simulink model "ex_longlat_kinematic"  (R2026a)
settings: Solver=VariableStepAuto
libraries: aerolibconvert2 x3
settings Model: Creator=doyeop  LastModifiedBy=doyeop

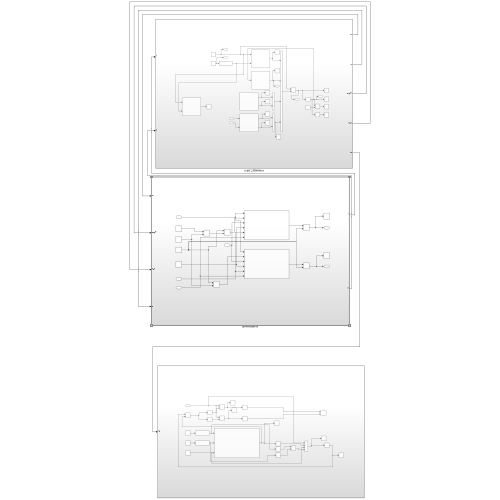
[thumbnail: Simulink's stored preview of the top-level diagram]
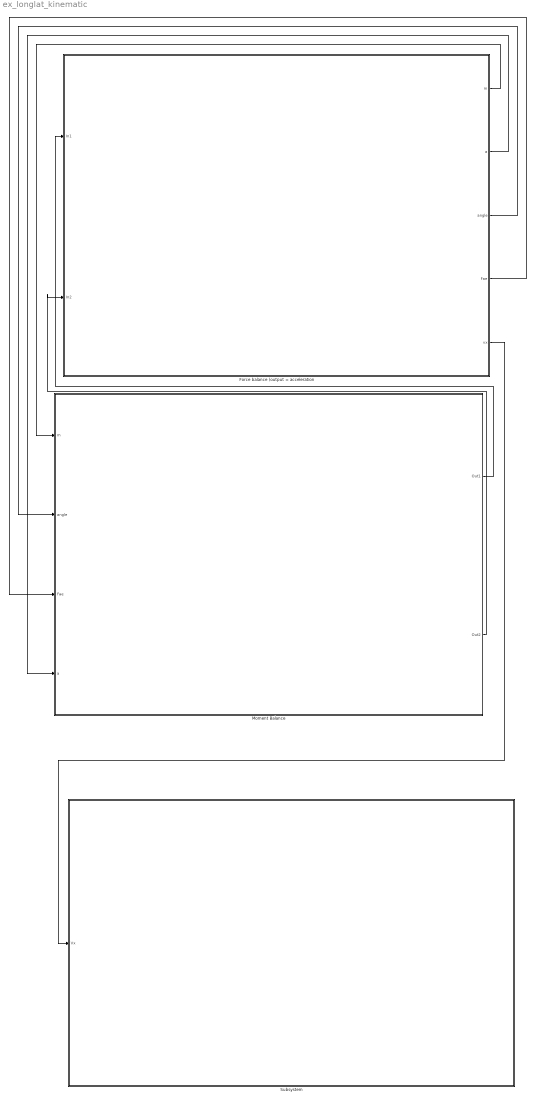
== system ex_longlat_kinematic ==
  Force balance (output = acceleration : Subsystem
  Moment Balance : Subsystem
  Subsystem : Subsystem
  wires:
  Force balance (output = acceleration/1(m) -> Moment Balance/1(m)
  Force balance (output = acceleration/2(a) -> Moment Balance/4(a)
  Force balance (output = acceleration/3(angle) -> Moment Balance/2(angle)
  Force balance (output = acceleration/4(Fae) -> Moment Balance/3(Fae)
  Moment Balance/1(Out1) -> Force balance (output = acceleration/1(In1)
  Moment Balance/2(Out2) -> Force balance (output = acceleration/2(In2)
  Force balance (output = acceleration/5(vx) -> Subsystem/1(Vx)

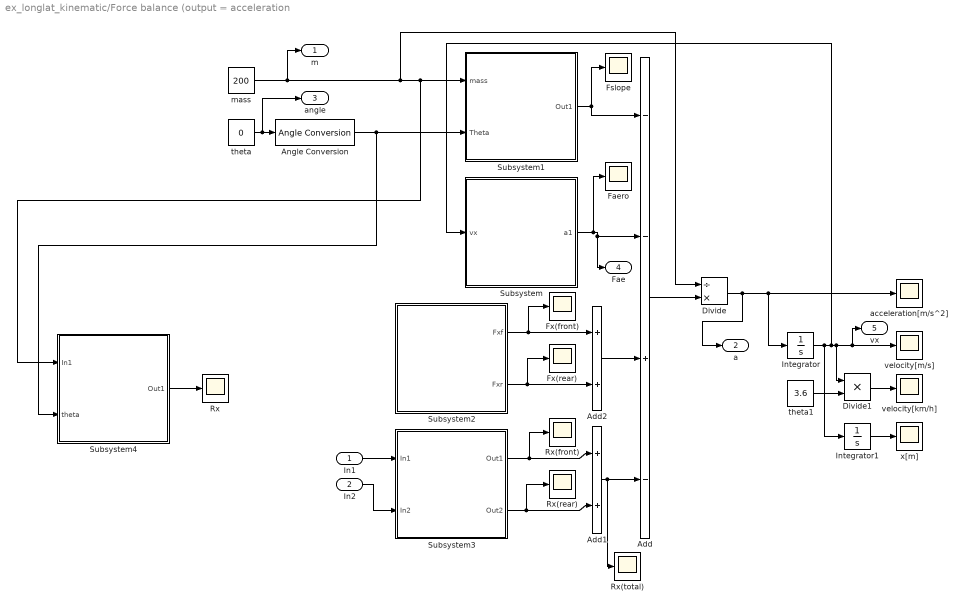
== system ex_longlat_kinematic/Force balance (output = acceleration ==
  In1 : Inport
  In2 : Inport  Port=2
  Add : Sum  Inputs=--+-
  Add1 : Sum
  Add2 : Sum
  Angle Conversion : aerolibconvert2/Angle Conversion  IU=deg  OU=rad
  Divide : Product  Inputs=/*
  Divide1 : Product  Inputs=**
  Faero : Scope
      settings: ActiveDisplayYMinimum=-21.806973838724872  ActiveDisplayYMaximum=245.93181269445461  DataLoggingVariableName=ScopeData4
  Fslope : Scope
      settings: ActiveDisplayYMinimum=467.68768501992645  ActiveDisplayYMaximum=4126.826484026702  DataLoggingVariableName=ScopeData3
  Fx(front) : Scope
      settings: ActiveDisplayYMinimum=-0.77322383064043154  ActiveDisplayYMaximum=0.91988628090500946  DataLoggingVariableName=ScopeData5
  Fx(rear) : Scope
      settings: ActiveDisplayYMinimum=-0.77322383064043154  ActiveDisplayYMaximum=0.91988628090500946  DataLoggingVariableName=ScopeData10
  Integrator : Integrator
  Integrator1 : Integrator
  Rx : Scope
      settings: ActiveDisplayYMinimum=21.392000000000003  ActiveDisplayYMaximum=41.392  DataLoggingVariableName=ScopeData6
  Rx(front) : Scope
      settings: ActiveDisplayYMinimum=-1  ActiveDisplayYMaximum=1  DataLoggingVariableName=ScopeData11
  Rx(rear) : Scope
      settings: ActiveDisplayYMinimum=-1  ActiveDisplayYMaximum=1  DataLoggingVariableName=ScopeData12
  Rx(total) : Scope
      settings: ActiveDisplayYMinimum=26.459225679325527  ActiveDisplayYMaximum=38.083177364358953  DataLoggingVariableName=ScopeData13
  Subsystem : Subsystem
  Subsystem1 : Subsystem
  Subsystem2 : Subsystem
  Subsystem3 : Subsystem
  Subsystem4 : Subsystem
  acceleration[m/s^2] : Scope
      settings: ActiveDisplayYMinimum=-1  ActiveDisplayYMaximum=1
  mass : Constant  Value=200  SampleTime=-1
  theta : Constant  Value=0  SampleTime=-1
  theta1 : Constant  Value=3.6  SampleTime=-1
  velocity[km/h] : Scope
      settings: ActiveDisplayYMinimum=-17.870991611228618  ActiveDisplayYMaximum=89.224414192347723  DataLoggingVariableName=ScopeData7
  velocity[m/s] : Scope
      settings: ActiveDisplayYMinimum=-1  ActiveDisplayYMaximum=1
  x[m] : Scope
      settings: ActiveDisplayYMinimum=-1  ActiveDisplayYMaximum=1  DataLoggingVariableName=ScopeData2
  m : Outport
  a : Outport  Port=2
  angle : Outport  Port=3
  Fae : Outport  Port=4
  vx : Outport  Port=5
  wires:
  Divide1/1 -> velocity[km/h]/1
  Subsystem/1(a1) -> Faero/1, Add/2, Fae/1
  Integrator1/1 -> x[m]/1
  Add/1 -> Divide/2
  Angle Conversion/1 -> Subsystem4/2(theta), Subsystem1/2(Theta)
  Divide/1 -> a/1, Integrator/1, acceleration[m/s^2]/1
  mass/1 -> m/1, Divide/1, Subsystem4/1(In1), Subsystem1/1(mass)
  Subsystem2/1(Fxf) -> Add2/1, Fx(front)/1
  theta1/1 -> Divide1/2
  Integrator/1 -> Integrator1/1, Subsystem/1(vx), Divide1/1, vx/1, velocity[m/s]/1
  Subsystem1/1(Out1) -> Fslope/1, Add/1
  Subsystem4/1(Out1) -> Rx/1
  theta/1 -> angle/1, Angle Conversion/1
  Subsystem2/2(Fxr) -> Fx(rear)/1, Add2/2
  In1/1 -> Subsystem3/1(In1)
  In2/1 -> Subsystem3/2(In2)
  Add1/1 -> Add/4, Rx(total)/1
  Subsystem3/2(Out2) -> Rx(rear)/1, Add1/2
  Subsystem3/1(Out1) -> Rx(front)/1, Add1/1
  Add2/1 -> Add/3

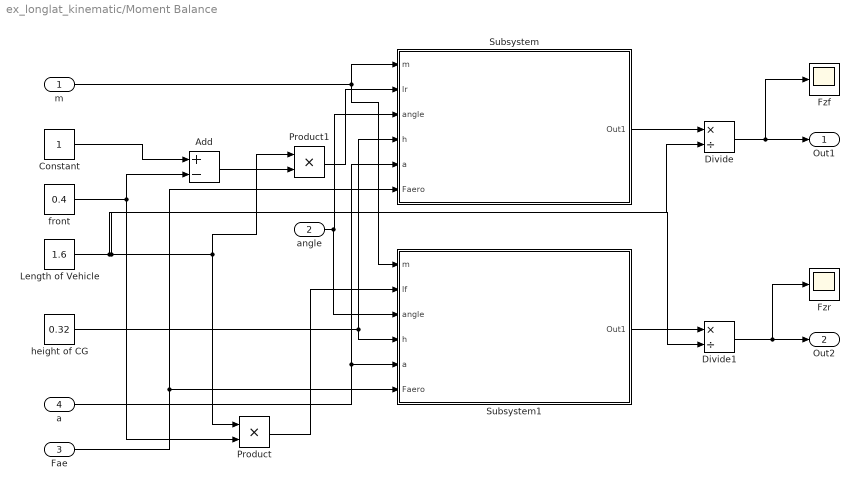
== system ex_longlat_kinematic/Moment Balance ==
  m : Inport
  angle : Inport  Port=2
  Fae : Inport  Port=3
  a : Inport  Port=4
  Add : Sum  Inputs=+-
  Constant : Constant
  Divide : Product  Inputs=*/
  Divide1 : Product  Inputs=*/
  Fzf : Scope
      settings: ActiveDisplayYMinimum=684.79999999999961  ActiveDisplayYMaximum=684.80000000000007  DataLoggingVariableName=ScopeData8
  Fzr : Scope
      settings: DataLoggingVariableName=ScopeData9
  Length of Vehicle : Constant  Value=1.6  SampleTime=-1
  Product : Product
  Product1 : Product
  Subsystem : Subsystem
  Subsystem1 : Subsystem
  front : Constant  Value=0.4  SampleTime=-1
  height of CG : Constant  Value=0.32
  Out1 : Outport
  Out2 : Outport  Port=2
  wires:
  m/1 -> Subsystem1/1(m), Subsystem/1(m)
  angle/1 -> Subsystem1/3(angle), Subsystem/3(angle)
  front/1 -> Product/2, Add/2
  Constant/1 -> Add/1
  Length of Vehicle/1 -> Divide/2, Divide1/2, Product1/1, Product/1
  Add/1 -> Product1/2
  Product1/1 -> Subsystem/2(lr)
  height of CG/1 -> Subsystem/4(h), Subsystem1/4(h)
  a/1 -> Subsystem1/5(a), Subsystem/5(a)
  Fae/1 -> Subsystem1/6(Faero), Subsystem/6(Faero)
  Subsystem/1(Out1) -> Divide/1
  Subsystem1/1(Out1) -> Divide1/1
  Product/1 -> Subsystem1/2(lf)
  Divide/1 -> Out1/1, Fzf/1
  Divide1/1 -> Fzr/1, Out2/1

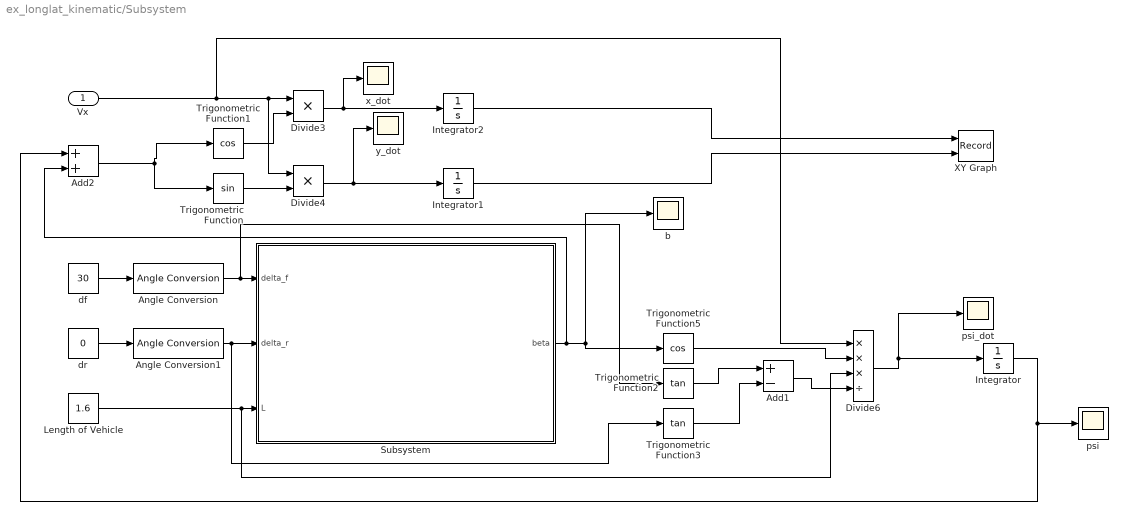
== system ex_longlat_kinematic/Subsystem ==
  Vx : Inport
  Add1 : Sum  Inputs=+-
  Add2 : Sum
  Angle Conversion : aerolibconvert2/Angle Conversion  IU=deg  OU=rad
  Angle Conversion1 : aerolibconvert2/Angle Conversion  IU=deg  OU=rad
  Divide3 : Product  Inputs=**
  Divide4 : Product  Inputs=**
  Divide6 : Product  Inputs=***/
  Integrator : Integrator
  Integrator1 : Integrator
  Integrator2 : Integrator
  Length of Vehicle : Constant  Value=1.6
  Subsystem : Subsystem
  Trigonometric Function : Trigonometry
  Trigonometric Function1 : Trigonometry  Operator=cos
  Trigonometric Function2 : Trigonometry  Operator=tan
  Trigonometric Function3 : Trigonometry  Operator=tan
  Trigonometric Function5 : Trigonometry  Operator=cos
  XY Graph : Record  NumPorts=2.0  FileSettingsInternal="{\"entries\":[{\"content\":{\"excelSettings\":{\"content\":{},\"type\":\"Streamout.ExcelSettings\"},\"parquetSettings\":{\"content\":{},\"type\":\"Streamout.ParquetSettings\"}},\"type\":\"Streamout.FileSettingStorage\",\"uuid\":\"\"}],\"packageUris\":[\"http:\\/\\/schema.mathworks.com\\/mf0\\/streamout_blocks\\/R2020a\"],\"version\":\"1.0\"}"  FrameSettings=[0, 0]  Layout=[1 1]  SignalsInternal="{\"entries\":[{\"content\":{\"signals\":[{\"content\":{\"blockPath\":[],\"dimensions\":[1],\"domain\":\"\",\"lineColor\":\"#a2142f\",\"plots\":[ 1 ],\"port\":1,\"sid\":[\"\"],\"signalID\":1,\"signalName\":\"Integrator2\"},\"type\":\"RecordBlkView.Signal\",\"uuid\":\"\"},{\"content\":{\"blockPath\":[],\"dimensions\":[1],\"domain\":\"\",\"lineColor\":\"#139fff\",\"plots\":[ 1 ],\"port\":2,\"sid\":[\"\"],\"signalID\":2,\"signalName\":\"Integrator1\"},\"type\":\"RecordBlkView.Signal\",\"uuid\":\"\"}]},\"type\":\"RecordBlkView.InputSignals\",\"uuid\":\"\"}],\"packageUris\":[\"http:\\/\\/schema.mathworks.com\\/mf0\\/streamout_blocks\\/R2020a\"],\"version\":\"1.0\"}"  VisualizationBindings="{\"xyplotplugin\":{\"info\":[{\"series\":[{\"bindingParametersList\":[{\"parameter\":\"X-Axis\",\"signalID\":1,\"signalName\":\"Integrator2\"},{\"parameter\":\"Y-Axis\",\"signalID\":2,\"signalName\":\"Integrator1\"}],\"seriesID\":0}],\"subplotID\":1}]}}"  CompatibilityTag=XY
  b : Scope
      settings: ActiveDisplayYMinimum=-1  ActiveDisplayYMaximum=1  DataLoggingVariableName=ScopeData14
  df : Constant  Value=30  SampleTime=-1
  dr : Constant  Value=0  SampleTime=-1
  psi : Scope
      settings: ActiveDisplayYMinimum=-238.30681397425238  ActiveDisplayYMaximum=2144.7613257682719  DataLoggingVariableName=ScopeData15
  psi_dot : Scope
      settings: ActiveDisplayYMinimum=-33.460316901439114  ActiveDisplayYMaximum=-7.0065127164247407  DataLoggingVariableName=ScopeData16
  x_dot : Scope
      settings: ActiveDisplayYMinimum=-1  ActiveDisplayYMaximum=1  DataLoggingVariableName=ScopeData17
  y_dot : Scope
      settings: ActiveDisplayYMinimum=-1  ActiveDisplayYMaximum=1  DataLoggingVariableName=ScopeData18
  wires:
  Add1/1 -> Divide6/4
  Integrator2/1 -> XY Graph/1
  Divide3/1 -> Integrator2/1, x_dot/1
  Subsystem/1(beta) -> Add2/2, b/1, Trigonometric Function5/1
  Trigonometric Function5/1 -> Divide6/2
  Trigonometric Function3/1 -> Add1/2
  Add2/1 -> Trigonometric Function1/1, Trigonometric Function/1
  Trigonometric Function1/1 -> Divide3/2
  Trigonometric Function/1 -> Divide4/2
  Divide4/1 -> Integrator1/1, y_dot/1
  Integrator/1 -> psi/1, Add2/1
  Integrator1/1 -> XY Graph/2
  Vx/1 -> Divide3/1, Divide4/1, Divide6/1
  Divide6/1 -> Integrator/1, psi_dot/1
  Trigonometric Function2/1 -> Add1/1
  Length of Vehicle/1 -> Divide6/3, Subsystem/3(L)
  df/1 -> Angle Conversion/1
  dr/1 -> Angle Conversion1/1
  Angle Conversion1/1 -> Subsystem/2(delta_r), Trigonometric Function3/1
  Angle Conversion/1 -> Trigonometric Function2/1, Subsystem/1(delta_f)

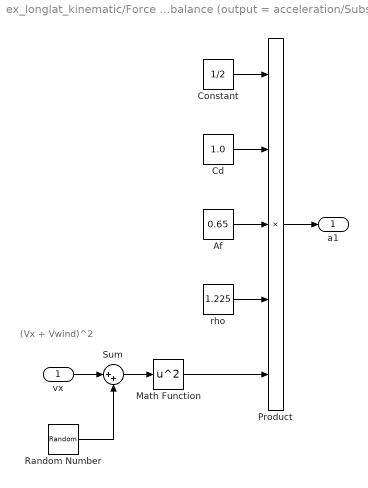
== system ex_longlat_kinematic/Force balance (output = acceleration/Subsystem ==
  note: (Vx + Vwind)^2
  vx : Inport
  Af : Constant  Value=0.65  SampleTime=-1
  Cd : Constant  Value=1.0  SampleTime=-1
  Constant : Constant  Value=1/2  SampleTime=-1
  Math Function : Math  Operator=square
  Product : Product  Inputs=5
  Random Number : RandomNumber  Mean=3  Variance=0.5^2  SampleTime=0.1
  Sum : Sum  Inputs=|++
  rho : Constant  Value=1.225  SampleTime=-1
  a1 : Outport
  wires:
  Cd/1 -> Product/2
  Af/1 -> Product/3
  Constant/1 -> Product/1
  rho/1 -> Product/4
  Random Number/1 -> Sum/2
  vx/1 -> Sum/1
  Sum/1 -> Math Function/1
  Math Function/1 -> Product/5
  Product/1 -> a1/1

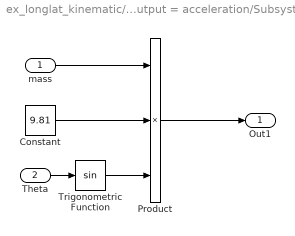
== system ex_longlat_kinematic/Force balance (output = acceleration/Subsystem1 ==
  mass : Inport
  Theta : Inport  Port=2
  Constant : Constant  Value=9.81  SampleTime=-1
  Product : Product  Inputs=3
  Trigonometric Function : Trigonometry
  Out1 : Outport
  wires:
  mass/1 -> Product/1
  Theta/1 -> Trigonometric Function/1
  Trigonometric Function/1 -> Product/3
  Constant/1 -> Product/2
  Product/1 -> Out1/1

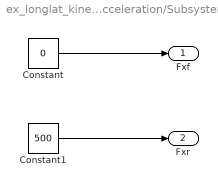
== system ex_longlat_kinematic/Force balance (output = acceleration/Subsystem2 ==
  Constant : Constant  Value=0  SampleTime=-1
  Constant1 : Constant  Value=500  SampleTime=-1
  Fxf : Outport
  Fxr : Outport  Port=2
  wires:
  Constant/1 -> Fxf/1
  Constant1/1 -> Fxr/1

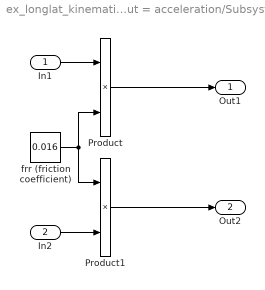
== system ex_longlat_kinematic/Force balance (output = acceleration/Subsystem3 ==
  In1 : Inport
  In2 : Inport  Port=2
  Product : Product
  Product1 : Product
  frr (friction coefficient) : Constant  Value=0.016  SampleTime=-1
  Out1 : Outport
  Out2 : Outport  Port=2
  wires:
  In1/1 -> Product/1
  frr (friction coefficient)/1 -> Product/2, Product1/1
  In2/1 -> Product1/2
  Product/1 -> Out1/1
  Product1/1 -> Out2/1

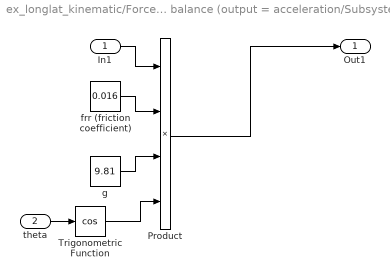
== system ex_longlat_kinematic/Force balance (output = acceleration/Subsystem4 ==
  In1 : Inport
  theta : Inport  Port=2
  Product : Product  Inputs=4
  Trigonometric Function : Trigonometry  Operator=cos
  frr (friction coefficient) : Constant  Value=0.016  SampleTime=-1
  g : Constant  Value=9.81  SampleTime=-1
  Out1 : Outport
  wires:
  In1/1 -> Product/1
  frr (friction coefficient)/1 -> Product/2
  g/1 -> Product/3
  theta/1 -> Trigonometric Function/1
  Product/1 -> Out1/1
  Trigonometric Function/1 -> Product/4

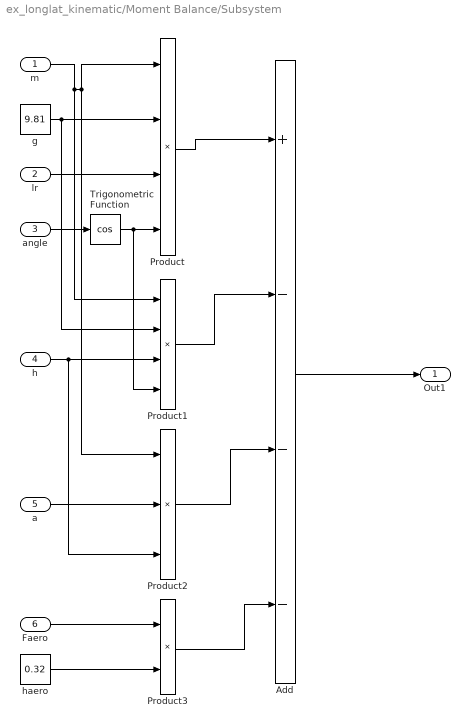
== system ex_longlat_kinematic/Moment Balance/Subsystem ==
  m : Inport
  lr : Inport  Port=2
  angle : Inport  Port=3
  h : Inport  Port=4
  a : Inport  Port=5
  Faero : Inport  Port=6
  Add : Sum  Inputs=+---
  Product : Product  Inputs=4
  Product1 : Product  Inputs=4
  Product2 : Product  Inputs=3
  Product3 : Product
  Trigonometric Function : Trigonometry  Operator=cos
  g : Constant  Value=9.81  SampleTime=-1
  haero : Constant  Value=0.32  SampleTime=-1
  Out1 : Outport
  wires:
  m/1 -> Product1/1, Product2/1, Product/1
  angle/1 -> Trigonometric Function/1
  g/1 -> Product1/2, Product/2
  lr/1 -> Product/3
  Trigonometric Function/1 -> Product1/4, Product/4
  a/1 -> Product2/2
  h/1 -> Product2/3, Product1/3
  haero/1 -> Product3/2
  Faero/1 -> Product3/1
  Product/1 -> Add/1
  Product1/1 -> Add/2
  Product2/1 -> Add/3
  Product3/1 -> Add/4
  Add/1 -> Out1/1

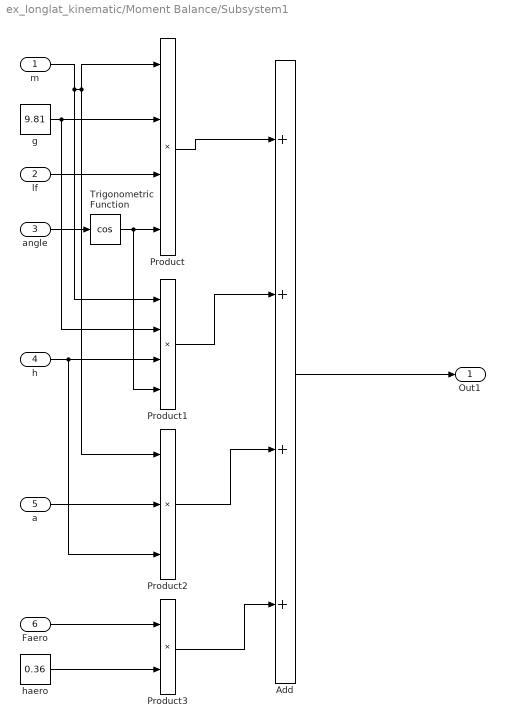
== system ex_longlat_kinematic/Moment Balance/Subsystem1 ==
  m : Inport
  lf : Inport  Port=2
  angle : Inport  Port=3
  h : Inport  Port=4
  a : Inport  Port=5
  Faero : Inport  Port=6
  Add : Sum  Inputs=++++
  Product : Product  Inputs=4
  Product1 : Product  Inputs=4
  Product2 : Product  Inputs=3
  Product3 : Product
  Trigonometric Function : Trigonometry  Operator=cos
  g : Constant  Value=9.81  SampleTime=-1
  haero : Constant  Value=0.36  SampleTime=-1
  Out1 : Outport
  wires:
  m/1 -> Product1/1, Product2/1, Product/1
  angle/1 -> Trigonometric Function/1
  g/1 -> Product1/2, Product/2
  lf/1 -> Product/3
  Trigonometric Function/1 -> Product1/4, Product/4
  a/1 -> Product2/2
  h/1 -> Product2/3, Product1/3
  haero/1 -> Product3/2
  Faero/1 -> Product3/1
  Product/1 -> Add/1
  Product1/1 -> Add/2
  Product2/1 -> Add/3
  Product3/1 -> Add/4
  Add/1 -> Out1/1

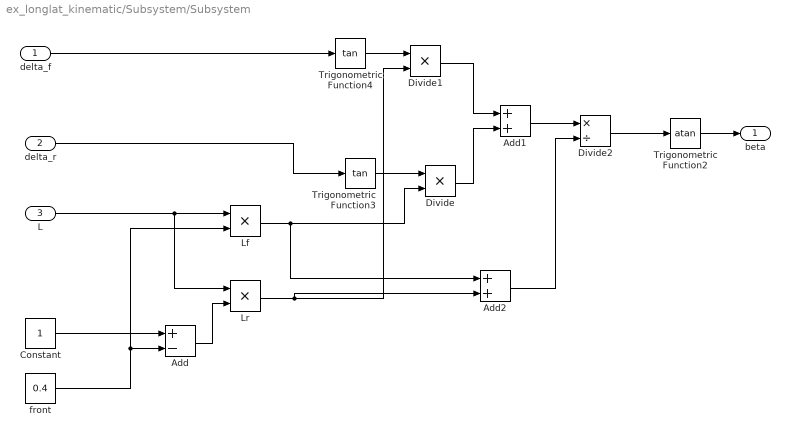
== system ex_longlat_kinematic/Subsystem/Subsystem ==
  delta_f : Inport
  delta_r : Inport  Port=2
  L : Inport  Port=3
  Add : Sum  Inputs=+-
  Add1 : Sum
  Add2 : Sum
  Constant : Constant  SampleTime=-1
  Divide : Product  Inputs=**
  Divide1 : Product  Inputs=**
  Divide2 : Product  Inputs=*/
  Lf : Product
  Lr : Product
  Trigonometric Function2 : Trigonometry  Operator=atan
  Trigonometric Function3 : Trigonometry  Operator=tan
  Trigonometric Function4 : Trigonometry  Operator=tan
  front : Constant  Value=0.4  SampleTime=-1
  beta : Outport
  wires:
  Trigonometric Function4/1 -> Divide1/1
  Lf/1 -> Add2/1, Divide/2
  Add1/1 -> Divide2/1
  Trigonometric Function2/1 -> beta/1
  front/1 -> Lf/2, Add/2
  Constant/1 -> Add/1
  delta_r/1 -> Trigonometric Function3/1
  Divide/1 -> Add1/2
  Trigonometric Function3/1 -> Divide/1
  Divide2/1 -> Trigonometric Function2/1
  L/1 -> Lr/1, Lf/1
  delta_f/1 -> Trigonometric Function4/1
  Lr/1 -> Add2/2, Divide1/2
  Add2/1 -> Divide2/2
  Divide1/1 -> Add1/1
  Add/1 -> Lr/2
